simulink model "test_instability"  (R2021b)
settings: Solver=FixedStepAuto  StartTime=0.0  StopTime=100  FixedStep=0.001  RelTol=1e-3
values from neighbouring files (symbols this model uses):
  mass = 1    [load_main.m]    (also in mod_k.m)
libraries: cstblocks x2
settings Model: Creator=chiara-s  LastModifiedBy=geriatronics
settings SolverCC: AlgebraicLoopSolver=TrustRegion
settings DebuggingCC: SFMachineParentedDataDiag=warning

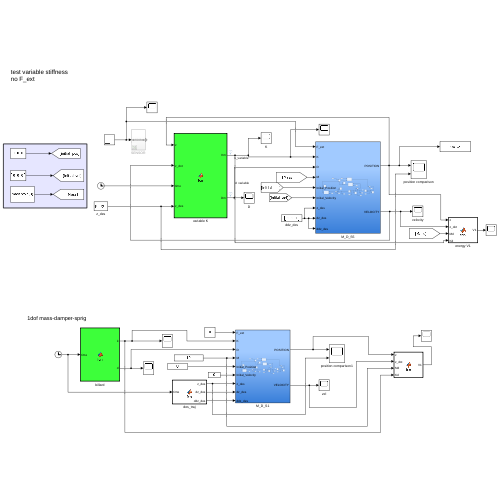
[thumbnail: Simulink's stored preview of the top-level diagram]
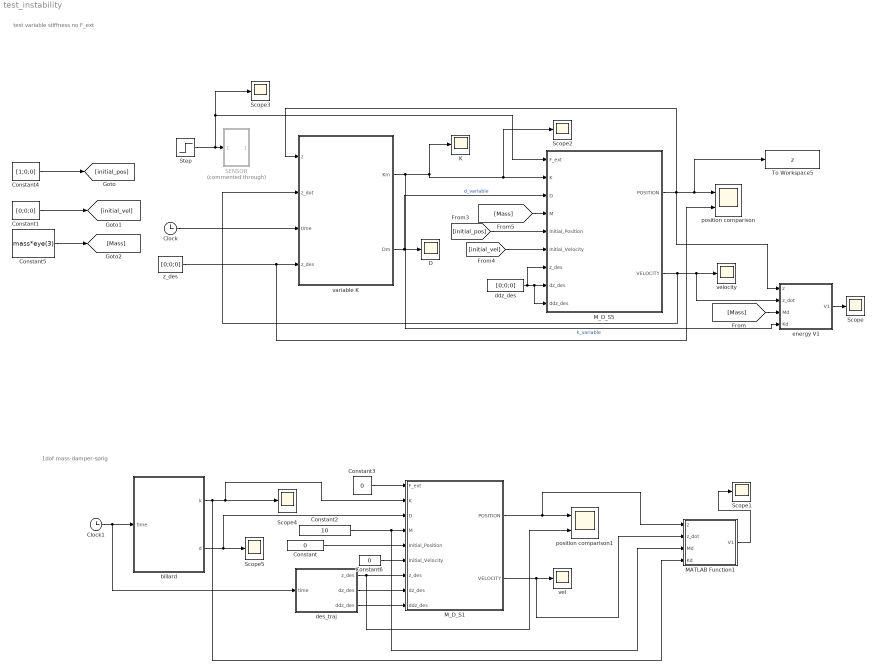
== system test_instability ==
  note: 1dof mass-damper-sprig
  note: test variable stiffness
      | no F_ext
  Clock : Clock
  Clock1 : Clock
  Constant : Constant  Value=0
  Constant1 : Constant  Value=[0;0;0]
  Constant2 : Constant  Value=10
  Constant3 : Constant  Value=0
  Constant4 : Constant  Value=[1;0;0]
  Constant5 : Constant  Value=mass*eye(3)
  Constant6 : Constant  Value=0
  D : Scope
  K : Scope
  MATLAB Function1 : MATLAB Function  TreatAsAtomicUnit=on
  M_D_S1 : Subsystem
  M_D_S5 : Subsystem
  SENSOR : Subsystem  Commented=through
  Scope{,1..5} (6 alike) : Scope
  Step : Step  Time=0  After=zeros(3,1)  SampleTime=0
  To Workspace5 : ToWorkspace  VariableName=z  SaveFormat=Structure With Time  SampleTime=-1
  billard : MATLAB Function  TreatAsAtomicUnit=on
  ddz_des : Constant  Value=[0;0;0]
  des_traj : MATLAB Function  TreatAsAtomicUnit=on
  energy V1 : MATLAB Function  TreatAsAtomicUnit=on
  position comparison : Scope  NumInputPorts=2
  position comparison1 : Scope  NumInputPorts=2
  variable K : MATLAB Function  TreatAsAtomicUnit=on
  vel : Scope
  velocity : Scope
  z_des : Constant  Value=[0;0;0]
  wires:
  variable K/2(Dm) -> M_D_S5/3(D), D/1  "d_variable"
  Constant1/1 -> [initial_vel]
  [Mass] -> M_D_S5/4(M)
  variable K/1(Km) -> energy V1/4(Kd), M_D_S5/2(K), Scope2/1, K/1  "k_variable"
  Constant4/1 -> [initial_pos]
  Clock/1 -> variable K/3(time)
  Constant5/1 -> [Mass]
  z_des/1 -> position comparison/2, variable K/4(z_des)
  Step/1 -> SENSOR/1(In1), Scope3/1, M_D_S5/1(F_ext)
  [initial_vel] -> M_D_S5/6(Initial_Velocity)
  M_D_S5/1(POSITION) -> energy V1/1(z), To Workspace5/1, position comparison/1, variable K/1(z)
  M_D_S5/2(VELOCITY) -> variable K/2(z_dot), energy V1/2(z_dot), velocity/1
  [Mass] -> energy V1/3(Md)
  energy V1/1(V1) -> Scope/1
  Constant/1 -> M_D_S1/5(Initial_Position)
  des_traj/1(z_des) -> position comparison1/2, M_D_S1/7(z_des)
  des_traj/2(dz_des) -> M_D_S1/8(dz_des)
  des_traj/3(ddz_des) -> M_D_S1/9(ddz_des)
  Constant2/1 -> MATLAB Function1/3(Md), M_D_S1/4(M)
  M_D_S1/1(POSITION) -> position comparison1/1, MATLAB Function1/1(z)
  M_D_S1/2(VELOCITY) -> MATLAB Function1/2(z_dot), vel/1
  MATLAB Function1/1(V1) -> Scope1/1
  billard/1(k) -> MATLAB Function1/4(Kd), M_D_S1/2(K), Scope4/1
  billard/2(d) -> Scope5/1, M_D_S1/3(D)
  [initial_pos] -> M_D_S5/5(Initial_Position)
  ddz_des/1 -> M_D_S5/7(z_des), M_D_S5/9(ddz_des), M_D_S5/8(dz_des)
  Clock1/1 -> des_traj/1(time), billard/1(time)
  Constant3/1 -> M_D_S1/1(F_ext)
  Constant6/1 -> M_D_S1/6(Initial_Velocity)

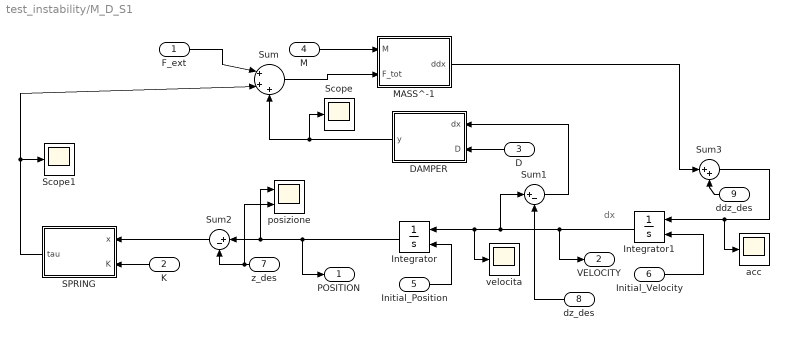
== system test_instability/M_D_S1 ==
  note: dx
  F_ext : Inport
  K : Inport  Port=2
  D : Inport  Port=3
  M : Inport  Port=4
  Initial_Position : Inport  Port=5
  Initial_Velocity : Inport  Port=6
  z_des : Inport  Port=7
  dz_des : Inport  Port=8
  ddz_des : Inport  Port=9
  DAMPER : MATLAB Function  TreatAsAtomicUnit=on
  Integrator : Integrator  InitialConditionSource=external
  Integrator1 : Integrator  InitialConditionSource=external
  MASS^-1 : MATLAB Function  TreatAsAtomicUnit=on
  SPRING : MATLAB Function  TreatAsAtomicUnit=on
  Scope : Scope
  Scope1 : Scope
  Sum : Sum  Inputs=|+++
  Sum1 : Sum  Inputs=|+-
  Sum2 : Sum  Inputs=|+-
  Sum3 : Sum  Inputs=|++
  acc : Scope
  posizione : Scope  NumInputPorts=2
  velocita : Scope
  POSITION : Outport
  VELOCITY : Outport  Port=2
  wires:
  Integrator1/1 -> velocita/1, Integrator/1, Sum1/1, VELOCITY/1
  SPRING/1(tau) -> Sum/2, Scope1/1
  Integrator/1 -> posizione/1, Sum2/1, POSITION/1
  DAMPER/1(y) -> Scope/1, Sum/3
  Sum/1 -> MASS^-1/2(F_tot)
  M/1 -> MASS^-1/1(M)
  D/1 -> DAMPER/2(D)
  K/1 -> SPRING/2(K)
  Initial_Velocity/1 -> Integrator1/2
  Initial_Position/1 -> Integrator/2
  z_des/1 -> posizione/2, Sum2/2
  Sum2/1 -> SPRING/1(x)
  MASS^-1/1(ddx) -> Sum3/1
  Sum1/1 -> DAMPER/1(dx)
  Sum3/1 -> acc/1, Integrator1/1
  dz_des/1 -> Sum1/2
  ddz_des/1 -> Sum3/2
  F_ext/1 -> Sum/1

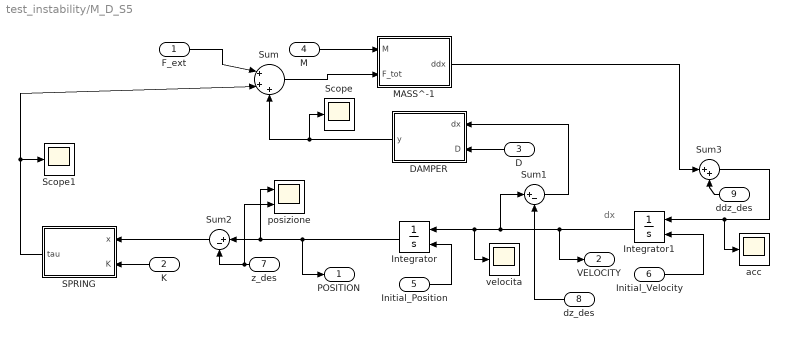
== system test_instability/M_D_S5 ==
  note: dx
  F_ext : Inport
  K : Inport  Port=2
  D : Inport  Port=3
  M : Inport  Port=4
  Initial_Position : Inport  Port=5
  Initial_Velocity : Inport  Port=6
  z_des : Inport  Port=7
  dz_des : Inport  Port=8
  ddz_des : Inport  Port=9
  DAMPER : MATLAB Function  TreatAsAtomicUnit=on
  Integrator : Integrator  InitialConditionSource=external
  Integrator1 : Integrator  InitialConditionSource=external
  MASS^-1 : MATLAB Function  TreatAsAtomicUnit=on
  SPRING : MATLAB Function  TreatAsAtomicUnit=on
  Scope : Scope
  Scope1 : Scope
  Sum : Sum  Inputs=|+++
  Sum1 : Sum  Inputs=|+-
  Sum2 : Sum  Inputs=|+-
  Sum3 : Sum  Inputs=|++
  acc : Scope
  posizione : Scope  NumInputPorts=2
  velocita : Scope
  POSITION : Outport
  VELOCITY : Outport  Port=2
  wires:
  Integrator1/1 -> velocita/1, Integrator/1, Sum1/1, VELOCITY/1
  SPRING/1(tau) -> Sum/2, Scope1/1
  Integrator/1 -> posizione/1, Sum2/1, POSITION/1
  DAMPER/1(y) -> Scope/1, Sum/3
  Sum/1 -> MASS^-1/2(F_tot)
  M/1 -> MASS^-1/1(M)
  D/1 -> DAMPER/2(D)
  K/1 -> SPRING/2(K)
  Initial_Velocity/1 -> Integrator1/2
  Initial_Position/1 -> Integrator/2
  z_des/1 -> posizione/2, Sum2/2
  Sum2/1 -> SPRING/1(x)
  MASS^-1/1(ddx) -> Sum3/1
  Sum1/1 -> DAMPER/1(dx)
  Sum3/1 -> acc/1, Integrator1/1
  dz_des/1 -> Sum1/2
  ddz_des/1 -> Sum3/2
  F_ext/1 -> Sum/1

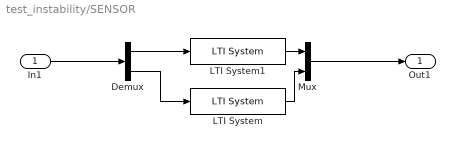
== system test_instability/SENSOR ==
  In1 : Inport
  Demux : Demux  Outputs=2
  LTI System : cstblocks/LTI System  sys=tf(200^2,[1 0.5*2*200 200^2])  IC=[]
  LTI System1 : cstblocks/LTI System  sys=tf(200^2,[1 0.5*2*200 200^2])  IC=[]
  Mux : Mux  Inputs=2
  Out1 : Outport
  wires:
  LTI System1/1 -> Mux/1
  Demux/1 -> LTI System1/1
  Demux/2 -> LTI System/1
  LTI System/1 -> Mux/2
  Mux/1 -> Out1/1
  In1/1 -> Demux/1

== matlab function test_instability/M_D_S5/DAMPER ==
  data: dx input; y output; D input
function y = fcn(dx, D)
y = - D*dx;
end

== matlab function test_instability/M_D_S5/MASS^-1 ==
  data: M input; ddx output; F_tot input
function ddx = fcn(M,F_tot)
ddx = (M^-1)*F_tot;


end

== matlab function test_instability/M_D_S5/SPRING ==
  data: x input; tau output; K input
function tau = fcn(x, K)
tau= -K*x;
end

== matlab function test_instability/billard ==
  settings: updateMethod=DISCRETE
  data: time input; k output; d output
function [k,d] = fcn(time)

%% Outputs
% Km            stiffness matrix
% Dm            damping matrix

%% Inputs
% time                   current simulation time
% mass                   mass scalar value 

%%unstable according to paper
k0 = 12; %N/m 
k = k0 + 10*sin(0.1*time);

%%try higher frequency 
% k0 = 12;
% k = k0 + 10*sin(1*time); 

d = 1; %N*s/m

% set final values 


end

== matlab function test_instability/energy V1 ==
  data: z input; V1 output; z_dot input; Md input; Kd input
function V1 = fcn(z,z_dot,Md,Kd)

V1 = 0.5*(z_dot'*Md*z_dot) + 0.5*(z'*Kd*z);

end

== matlab function test_instability/M_D_S1/DAMPER ==
  data: dx input; y output; D input
function y = fcn(dx, D)
y = - D*dx;
end

== matlab function test_instability/M_D_S1/MASS^-1 ==
  data: M input; ddx output; F_tot input
function ddx = fcn(M,F_tot)
ddx = (M^-1)*F_tot;


end

== matlab function test_instability/M_D_S1/SPRING ==
  data: x input; tau output; K input
function tau = fcn(x, K)
tau= -K*x;
end

== matlab function test_instability/des_traj ==
  data: time input; z_des output; dz_des output; ddz_des output
function [z_des,dz_des,ddz_des] = fcn(time)

z_des = 10*sin(0.1*time);
dz_des = cos(0.1*time);
ddz_des = -0.1*sin(0.1*time);

end

== matlab function test_instability/MATLAB Function1 ==
  data: z input; V1 output; z_dot input; Md input; Kd input
function V1 = fcn(z,z_dot,Md,Kd)

V1 = 0.5*(Md*z_dot^2) + 0.5*(Kd*z^2);

end

== matlab function test_instability/variable K ==
  settings: updateMethod=DISCRETE
  data: Km output; Dm output; z input; z_dot input; time input; z_des input; mass parameter
function [Km,Dm] = fcn(z, z_dot, time, z_des, mass)

%% Description
% decrease k after contact is sensed to limit the interaction force

%% Outputs
% Km            stiffness matrix
% Dm            damping matrix

%% Inputs
% time                   current simulation time
% mass                   mass scalar value 
% z_des, dz_des,ddz_des  desired trajectory
% z                      current position
% dz                     current velocity
% F_max         estimated force disturbances
% e_max         maximum steady-state error

persistent kx0 ky0 kz0 dx dy dz t_changex t_changey t_changez kx ky kz faraway_x faraway_y faraway_z kchange_x kchange_y kchange_z

% time of last stiffness update
if isempty(t_changex)
    t_changex = 0;
end
if isempty(t_changey)
    t_changey = 0;
end
if isempty(t_changez)
    t_changez = 0;
end

% initialization of k and d 
if isempty(kx0)
   kx0 = 300; 
end
if isempty(ky0)
   ky0 = 300;
end

if isempty(kz0)
   kz0 = 300;
end

if isempty(dx)
    dx = sqrt(4*kx0*mass)/10;
end
if isempty(dy)
    dy = sqrt(4*ky0*mass)/10;
end
if isempty(dz)
    dz = sqrt(4*kz0*mass)/10;
end


if isempty(kx) 
    kx = kx0;
end
if isempty(ky)
    ky = ky0;
end

if isempty(kz)
    kz = kz0;
end

if isempty(faraway_x)
    faraway_x = 10;
end
if isempty(faraway_y)
    faraway_y = 10;
end
if isempty(faraway_z)
    faraway_z = 10;
end

if isempty(kchange_x)
    kchange_x = kx0;
end
if isempty(kchange_y)
    kchange_y = ky0;
end
if isempty(kchange_z)
    kchange_z = kz0;
end

%% discontinuous instability
%       kx = kx0 - (kx0/2)*sign(z_dot(1)*(z(1)-z_des(1)));                      %instability
%       ky = ky0 - (ky0/2)*sign(z_dot(2)*(z(2)-z_des(2)));

%% continuous instability

t = 10000;    % slope

% x-axis
if sign(z_dot(1)*(z(1)-z_des(1))) > 0 
    if faraway_x == 10
        faraway_x = 1;
    elseif faraway_x == 0 
        t_changex = time; 
        faraway_x = 1;
        kchange_x = kx;
    end
    kfx = kx0 - kx0/2;
    k_dotx = -t;
    k_tempx = kchange_x + k_dotx*(time - t_changex);
    if k_tempx < kfx
        kx = kfx;
    else
        kx = k_tempx;
    end
else 
    if faraway_x == 10
        faraway_x = 0;
    elseif faraway_x == 1
        t_changex = time;
        faraway_x = 0;
        kchange_x = kx;
    end
    kfx = kx0 + kx0/2;
    k_dotx = t;
    k_tempx = kchange_x + k_dotx*(time - t_changex);
    if k_tempx > kfx
        kx = kfx;
    else
        kx = k_tempx;
    end
end

% y-axis
if sign(z_dot(2)*(z(2)-z_des(2))) > 0 
    if faraway_y == 10
        faraway_y = 1;
    elseif faraway_y == 0 
        t_changey = time; 
        faraway_y = 1;
        kchange_y = ky;
    end
    kfy = ky0 - ky0/2;
    k_doty = -t;
    k_tempy = kchange_y + k_doty*(time - t_changey);
    if k_tempy < kfy
        ky = kfy;
    else
        ky = k_tempy;
    end
else 
    if faraway_y == 10
        faraway_y = 0;
    elseif faraway_y == 1
        t_changey = time;
        faraway_y = 0;
        kchange_y = ky;
    end
    kfy = ky0 + ky0/2;
    k_doty = t;
    k_tempy = kchange_y + k_doty*(time - t_changey);
    if k_tempy > kfy
        ky = kfy;
    else
        ky = k_tempy;
    end
end


% z-axis
if sign(z_dot(3)*(z(3)-z_des(3))) > 0 
    if faraway_z == 10
        faraway_z = 1;
    elseif faraway_z == 0 
        t_changez = time; 
        faraway_z = 1;
        kchange_z = kz;
    end
    kfz = kz0 - kz0/2;
    k_dotz = -t;
    k_tempz = kchange_z + k_dotz*(time - t_changez);
    if k_tempz < kfz
        kz = kfz;
    else
        kz = k_tempz;
    end
else 
    if faraway_z == 10
        faraway_z = 0;
    elseif faraway_z == 1
        t_changez = time;
        faraway_z = 0;
        kchange_z = kz;
    end
    kfz = kz0 + kz0/2;
    k_dotz = t;
    k_tempz = kchange_z + k_dotz*(time - t_changez);
    if k_tempz > kfz
        kz = kfz;
    else
        kz = k_tempz;
    end
end


% set final values 
Dm = diag([dx,dy,dz]);
Km = diag([kx,ky,kz]);

end
